simulink model "Simple_DualPortRAM_Ex1"  (R2025a)
settings: Solver=VariableStepAuto  StartTime=0.0  StopTime=1e3  RelTol=1e-3
libraries: hdlBasic x6, hdlsllib x3, hdlUtilities x1, dspobslib x1, dspsrcs4 x1, vmcUtilities x1
settings Model: Creator=sdegala  LastModifiedBy=robg

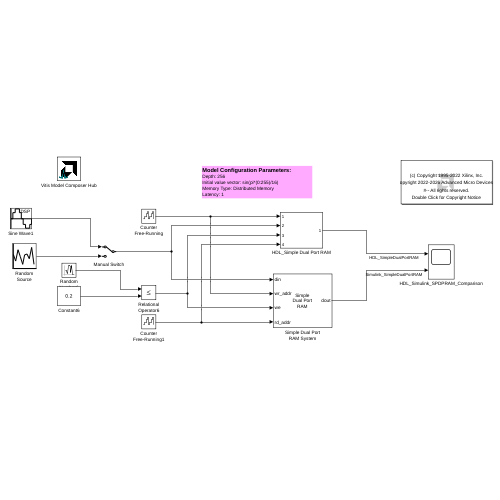
[thumbnail: Simulink's stored preview of the top-level diagram]
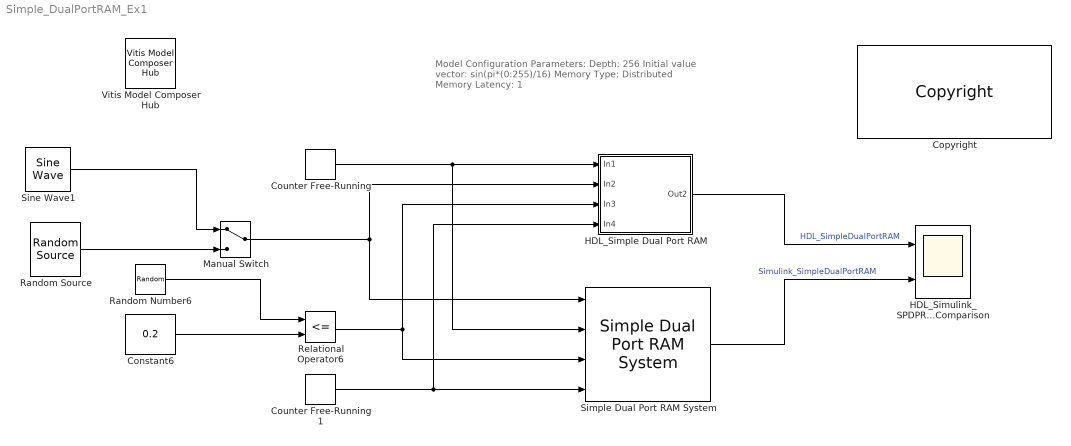
== system Simple_DualPortRAM_Ex1 ==
  note: Model Configuration Parameters:
      | Depth: 256
      | Initial value vector: sin(pi*(0:255)/16)
      | Memory Type: Distributed Memory
      | Latency: 1
  Constant6 : Constant  Value=0.2
  Copyright : hdlUtilities/Copyright  copyrighttext="(c) Copyright 1995-2022 Xilinx, Inc. <br>(c) Copyright 2022-2026 Advanced Micro Devices, Inc. All rights reserved.<br><br>This document  contains proprietary, confidential information that may be used, copied and/or disclosed only as authorized by a valid licensing agreement with Advanced Micro Devices, Inc. This copyright notice must be retained on all authorized copies.<br><br> This code is provided \"as is\". Advanced Micro Devices, Inc. makes, and the end user receives, no warranties or conditions, express, implied, statutory or otherwise, and Advanced Micro Devices, Inc. specifically disclaims any implied warranties of merchantability, <br>non-infringement, or fitness for a particular purpose."  block_type=copyright
  Counter Free-Running : hdlsllib/Sources/Counter Free-Running  NumBits=8  tsamp=2
  Counter Free-Running1 : hdlsllib/Sources/Counter Free-Running  NumBits=8  tsamp=4
  HDL_Simple Dual Port RAM : Subsystem
  HDL_Simulink_SPDPRAM_Comparison : Scope  NumInputPorts=2
      settings: ActiveDisplayYMinimum=-5  ActiveDisplayYMaximum=5
  Manual Switch : ManualSwitch
  Random Number6 : RandomNumber  Seed=65536  SampleTime=0
  Random Source : dspobslib/Random Source  SrcType=Uniform  NormMethod=Ziggurat  CltLength=12  MinVal=0  MaxVal=1  MeanVal=0  VarVal=1  RepMode=Specify seed  rawSeed=1  IsInherit=off  SampMode=Discrete  SampTime=1  SampFrame=1  DataType=Double  OutComplex=Real  OutputFrames=on
  Relational Operator6 : RelationalOperator  Operator=<=
  Simple Dual Port RAM System : hdlsllib/HDL RAMs/Simple Dual Port RAM System  RAMType=Simple dual port  AsyncRead=off  WriteOutputValue=New data  RAMInitialValue=sin(pi*(0:255)/16)  allowBusInputs=off  WritesHaveOutput=on  NumReads=0  NumWrites=1  SimulateUsing=Code generation  ModelRAMDelay=on  VectorAccess=Parallel
  Sine Wave1 : dspsrcs4/Sine Wave  Amplitude=1  Frequency=0.15  Phase=0  SampleMode=Discrete  OutComplex=Real  CompMethod=Trigonometric fcn  TableSize=Speed  SampleTime=1  SamplesPerFrame=1  ResetState=Restart at time zero  OutputFrames=off  dataType=double  wordLen=16  udDataType=sfix(16)  fracBitsMode=Best precision  numFracBits=15  OutDataTypeStr=double  LastOutDataTypeStr=double
  Vitis Model Composer Hub : vmcUtilities/Vitis Model Composer Hub  Tag=genX  CodeGeneration=off  SubsystemName=HDL_Simple Dual Port RAM  StartColumn=1  NumberOfColumns=1  TargetDirectory=./code  exportDesign=off  analyzeDesign=off  validateDesignOnHw=off  ExportType=System Generator  IpVendor=xilinx.com  IpLibrary=hls  IpVersion=1.0  IpHWLanguage=Verilog  AieCompilerOptions={}  AieSimulatorOptions={}  CreateTestbench=off  TestbenchStackSize=10  RunRtlSim=off  RunCSim=off  RunAieSim=off  enableSimulationTimeout=on  enableGraphIterations=on  AieSimTimeout=50000  AieGraphIterations=-1  RunAieSimProfiling=off  LaunchVitisAnalyzer=off  PlotOutput=off  RunX86Sim=off  X86SimTimeout=10  GenHwImage=off  GenLibadfXo=on  GenHwValidationCode=off  PlatformType=Not Specified  HwSystemType=Baremetal  HwValidationTarget=hw  ProjDevice=xcvu9p-fsgd2104-3-e  ProjDevicePart=xcvu9p-fsgd2104-3-e  SamplePeriod=-1  ClockFrequency=200  DataPathParallelism=1  xilinxfamily=virtexuplus  part=xcvu9p  speed=-3-e  package=fsgd2104  directory=./netlist/ip/HDL_Simple_Dual_Port_RAM/src  testbench=off  incr_netlist=off  synthesis_tool=Vivado  clock_wrapper=Clock Enables  dbl_ovrd=According to Block Masks  dcm_input_clock_period=10  sysclk_period=10  simulink_period=1  eval_field=0  LogFileName=''  NThreads=4
  wires:
  Random Number6/1 -> Relational Operator6/1
  HDL_Simple Dual Port RAM/1(Out2) -> HDL_Simulink_SPDPRAM_Comparison/1  "HDL_SimpleDualPortRAM"
  Constant6/1 -> Relational Operator6/2
  Relational Operator6/1 -> Simple Dual Port RAM System/3, HDL_Simple Dual Port RAM/3(In3)
  Counter Free-Running/1 -> Simple Dual Port RAM System/2, HDL_Simple Dual Port RAM/1(In1)
  Counter Free-Running1/1 -> HDL_Simple Dual Port RAM/4(In4), Simple Dual Port RAM System/4
  Simple Dual Port RAM System/1 -> HDL_Simulink_SPDPRAM_Comparison/2  "Simulink_SimpleDualPortRAM"
  Sine Wave1/1 -> Manual Switch/1
  Manual Switch/1 -> Simple Dual Port RAM System/1, HDL_Simple Dual Port RAM/2(In2)
  Random Source/1 -> Manual Switch/2

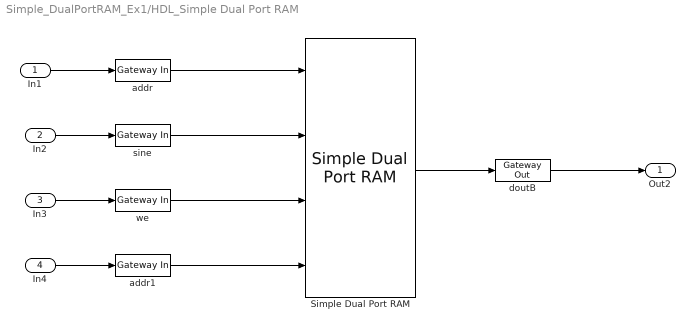
== system Simple_DualPortRAM_Ex1/HDL_Simple Dual Port RAM ==
  In1 : Inport
  In2 : Inport  Port=2
  In3 : Inport  Port=3
  In4 : Inport  Port=4
  Simple Dual Port RAM : hdlBasic/Simple Dual Port RAM  depth=256  initVector=sin(pi*(0:255)/16)  distributed_mem=Distributed memory  init_b=0  rst_b=off  en_a=off  en_b=off  latency=1  write_mode_B=Read After Write  optimize=Speed  explicit_period=[]  period=[]  simulation_type=fast_sim  XmcBlockStatus=1  maskContainerNames=tabcontainer1  block_type=sdpram  block_config=sysgen:Sdpram_config
      settings: infoedit=[]
  addr : hdlBasic/Gateway In  gui_display_data_type=Fixed-point  arith_type=Unsigned  n_bits=8  bin_pt=0  preci_type=Single  exp_width=8  frac_width=24  rows=1  columns=1  quantization="Round  (unbiased: +/- Inf)"  overflow=Saturate  period=1  UseAsADC=off  ADCChannel='1'  interface=None  automatic_assignment=on  address_offset=hex2dec('00')  intf_name=''  intf_description=''  default_value=0  timing_constraint=None  locs_specified=off  LOCs={}  io_standard={}  inherit_from_input=off  hdl_port=on  XmcBlockStatus=1  maskContainerNames=group4  block_type=gatewayin  block_config=sysgen:gateway_in_config  block_width_w=590  block_height_w=620  block_width=640  block_height=850
  addr1 : hdlBasic/Gateway In  gui_display_data_type=Fixed-point  arith_type=Unsigned  n_bits=8  bin_pt=0  preci_type=Single  exp_width=8  frac_width=24  rows=1  columns=1  quantization="Round  (unbiased: +/- Inf)"  overflow=Saturate  period=1  UseAsADC=off  ADCChannel='1'  interface=None  automatic_assignment=on  address_offset=hex2dec('00')  intf_name=''  intf_description=''  default_value=0  timing_constraint=None  locs_specified=off  LOCs={}  io_standard={}  inherit_from_input=off  hdl_port=on  XmcBlockStatus=1  maskContainerNames=group4  block_type=gatewayin  block_config=sysgen:gateway_in_config  block_width_w=590  block_height_w=620  block_width=640  block_height=850
  doutB : hdlBasic/Gateway Out  inherit_from_input=off  bool_to_boolean=off  hdl_port=on  rows=1  columns=1  UseAsDAC=off  DACChannel='1'  interface=None  automatic_assignment=on  address_offset=hex2dec('00')  intf_name=''  intf_description=''  timing_constraint=None  locs_specified=off  LOCs={}  io_standard={}  XmcBlockStatus=1  maskContainerNames=group4  block_type=gatewayout  block_config=sysgen:gateway_out_config  block_width_w=590  block_height_w=620  block_width=620  block_height=750
  sine : hdlBasic/Gateway In  gui_display_data_type=Fixed-point  arith_type=Signed (2's comp)  n_bits=8  bin_pt=6  preci_type=Single  exp_width=8  frac_width=24  rows=1  columns=1  quantization="Round  (unbiased: +/- Inf)"  overflow=Saturate  period=1  UseAsADC=off  ADCChannel='1'  interface=None  automatic_assignment=on  address_offset=hex2dec('00')  intf_name=''  intf_description=''  default_value=0  timing_constraint=None  locs_specified=off  LOCs={}  io_standard={}  inherit_from_input=off  hdl_port=on  XmcBlockStatus=1  maskContainerNames=group4  block_type=gatewayin  block_config=sysgen:gateway_in_config  block_width_w=590  block_height_w=620  block_width=640  block_height=850
  we : hdlBasic/Gateway In  gui_display_data_type=Boolean  arith_type=Boolean  n_bits=1  bin_pt=0  preci_type=Single  exp_width=8  frac_width=24  rows=1  columns=1  quantization="Round  (unbiased: +/- Inf)"  overflow=Saturate  period=1  UseAsADC=off  ADCChannel='1'  interface=None  automatic_assignment=on  address_offset=hex2dec('00')  intf_name=''  intf_description=''  default_value=0  timing_constraint=None  locs_specified=off  LOCs={}  io_standard={}  inherit_from_input=off  hdl_port=on  XmcBlockStatus=1  maskContainerNames=group4  block_type=gatewayin  block_config=sysgen:gateway_in_config  block_width_w=590  block_height_w=620  block_width=640  block_height=850
  Out2 : Outport
  wires:
  Simple Dual Port RAM/1 -> doutB/1
  addr/1 -> Simple Dual Port RAM/1
  In2/1 -> sine/1
  In4/1 -> addr1/1
  doutB/1 -> Out2/1
  In1/1 -> addr/1
  In3/1 -> we/1
  addr1/1 -> Simple Dual Port RAM/4
  we/1 -> Simple Dual Port RAM/3
  sine/1 -> Simple Dual Port RAM/2
